simulink model "practicatressimulink"  (R2024b)
settings: Solver=VariableStepAuto  StartTime=0.0  StopTime=15  RelTol=1e-3
InitFcn:
  | m1=290;
  | b1=1000;
  | m2=59;
  | k1=16182;
  | f=0;
  | t=15;
  | k2=19000;

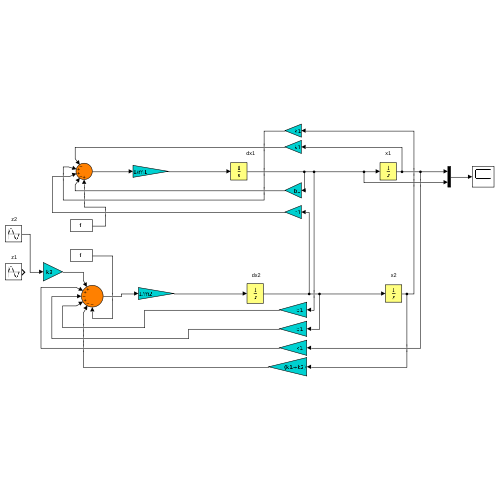
[thumbnail: Simulink's stored preview of the top-level diagram]
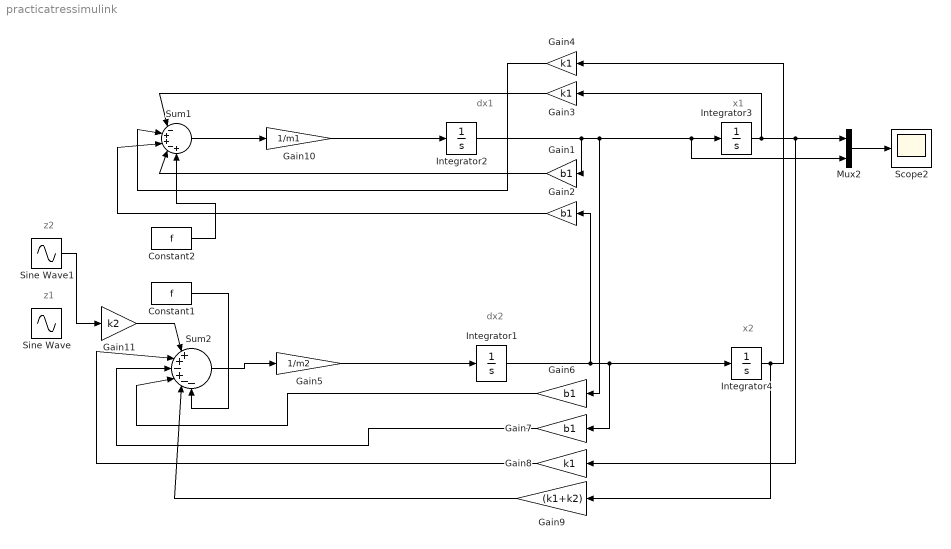
== system practicatressimulink ==
  note: z1
  note: dx1
  note: x1
  note: x2
  note: dx2
  note: z2
  Constant1 : Constant  Value=f
  Constant2 : Constant  Value=f
  Gain{1..2,6..7} (4 alike) : Gain  Gain=b1
  Gain10 : Gain  Gain=1/m1
  Gain11 : Gain  Gain=k2
  Gain3 : Gain  Gain=k1
  Gain4 : Gain  Gain=k1
  Gain5 : Gain  Gain=1/m2
  Gain8 : Gain  Gain=k1
  Gain9 : Gain  Gain=(k1+k2)
  Integrator{1..4} (4 alike) : Integrator
  Mux2 : Mux  Inputs=2
  Scope2 : Scope
  Sine Wave : Sin  Amplitude=0.05  Frequency=0.5 * pi  SampleTime=0
  Sine Wave1 : Sin  Amplitude=0.05  Frequency=20 * pi  SampleTime=0
  Sum1 : Sum  Inputs=|-++-+
  Sum2 : Sum  Inputs=|++-+--
  wires:
  Gain10/1 -> Integrator2/1
  Mux2/1 -> Scope2/1
  Integrator3/1 -> Gain3/1, Gain8/1, Mux2/1
  Sum1/1 -> Gain10/1
  Integrator4/1 -> Gain9/1, Gain4/1
  Sum2/1 -> Gain5/1
  Gain1/1 -> Sum1/4
  Integrator1/1 -> Gain2/1, Gain7/1, Integrator4/1
  Gain2/1 -> Sum1/3
  Gain3/1 -> Sum1/1
  Gain4/1 -> Sum1/2
  Gain5/1 -> Integrator1/1
  Gain11/1 -> Sum2/1
  Gain6/1 -> Sum2/4
  Gain7/1 -> Sum2/3
  Gain8/1 -> Sum2/2
  Integrator2/1 -> Gain1/1, Gain6/1, Mux2/2, Integrator3/1
  Gain9/1 -> Sum2/5
  Constant1/1 -> Sum2/6
  Constant2/1 -> Sum1/5
  Sine Wave1/1 -> Gain11/1
